simulink model "State_Space_Discrete"  (Simulink 8.0)
settings: Solver=ode45  StartTime=0.0  StopTime=10.0  RelTol=1e-3
undefined symbols (not defined in the file or in its folder): Ac, Ad, Bc, Bd
settings Model: Creator=Faradars  LastModifiedBy=Faradars

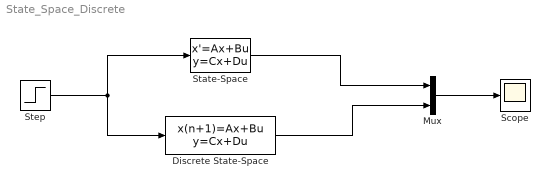
== system State_Space_Discrete ==
  Discrete State-Space : DiscreteStateSpace  A=Ad  B=Bd  C=[0 1]  D=0  SampleTime=0.1
  Mux : Mux  Inputs=2
  Scope : Scope
  State-Space : StateSpace  A=Ac  B=Bc  C=[0 1]  D=0
  Step : Step  SampleTime=0.1
  wires:
  Mux/1 -> Scope/1
  Discrete State-Space/1 -> Mux/2
  State-Space/1 -> Mux/1
  Step/1 -> State-Space/1, Discrete State-Space/1
